simulink model "RotationalSolarPanelControl"  (R2022b)
settings: Solver=VariableStepAuto  StartTime=0.0  StopTime=15  RelTol=1e-3
undefined symbols (not defined in the file): J, Kd, Kf, Kg, Kt, R
libraries: slpidlib x1
settings Model: Creator=juan.moreira  LastModifiedBy=jprmj
settings ModelReferenceCC: EnableRefExpFcnMdlSchedulingChecks=on

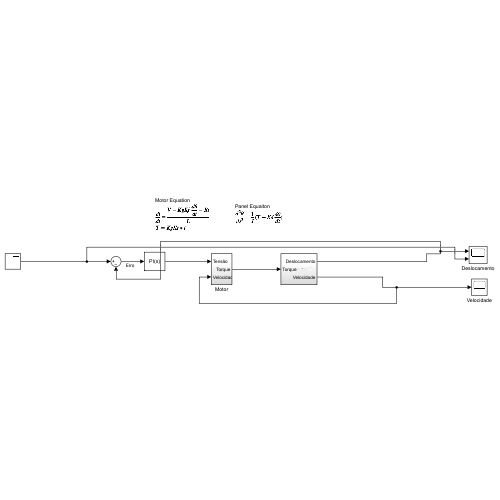
[thumbnail: Simulink's stored preview of the top-level diagram]
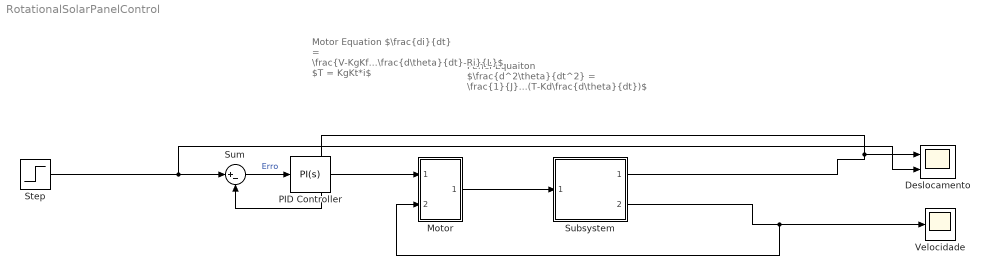
== system RotationalSolarPanelControl ==
  note: Panel Equaiton
      | $\frac{d^2\theta}{dt^2} = \frac{1}{J}(T-Kd\frac{d\theta}{dt})$
  note: Motor Equation
      | $\frac{di}{dt} = \frac{V-KgKf\frac{d\theta}{dt}-Ri}{L}$
      | $T = KgKt*i$
  Deslocamento : Scope  NumInputPorts=2
  Motor : Subsystem
  PID Controller : slpidlib/PID Controller  Controller=PI  Form=Parallel  TimeDomain=Continuous-time  UseExternalTs=off  SampleTime=-1  IntegratorMethod=Forward Euler  FilterMethod=Forward Euler  ControllerParametersSource=internal  P=180  I=140  UseKiTs=off  D=0  N=100  UseFilter=on  TunerSelectOption=Transfer Function Based (PID Tuner App)  InitialConditionSource=internal  InitialConditionForIntegrator=0  InitialConditionForFilter=0  DifferentiatorICPrevScaledInput=0  ExternalReset=none  TrackingMode=off  Kt=1  LimitOutput=off  SatLimitsSource=internal  UpperSaturationLimit=inf  LowerSaturationLimit=-inf  LinearizeAsGain=on  AntiWindupMode=none  Kb=1  LimitIntegrator=off  UpperIntegratorSaturationLimit=inf  LowerIntegratorSaturationLimit=-inf  POutMin=[]  POutMax=[]  IOutMin=[]  IOutMax=[]  DOutMin=[]  DOutMax=[]  NOutMin=[]  NOutMax=[]  SumOutMin=[]  SumOutMax=[]  SaturationOutMin=[]  SaturationOutMax=[]  PParamMin=[]  PParamMax=[]  IParamMin=[]  IParamMax=[]  DParamMin=[]  DParamMax=[]  NParamMin=[]  NParamMax=[]  KbParamMin=[]  KbParamMax=[]  KtParamMin=[]  KtParamMax=[]  KbOutMin=[]  KbOutMax=[]  KtOutMin=[]  KtOutMax=[]  IntegratorOutMin=[]  IntegratorOutMax=[]  FilterOutMin=[]  FilterOutMax=[]  SumI1OutMin=[]  SumI1OutMax=[]  SumI2OutMin=[]  SumI2OutMax=[]  SumI3OutMin=[]  SumI3OutMax=[]  SumI4OutMin=[]  SumI4OutMax=[]  SumDOutMin=[]  SumDOutMax=[]  DifferentiatorOutMin=[]  DifferentiatorOutMax=[]  FilterDiffOutCoefMin=[]  FilterDiffOutCoefMax=[]  ReciprocalOutMin=[]  ReciprocalOutMax=[]  SumDenOutMin=[]  SumDenOutMax=[]  SumNumOutMin=[]  SumNumOutMax=[]  DivideOutMin=[]  DivideOutMax=[]  UdiffTsProdOutMin=[]  UdiffTsProdOutMax=[]  NTsProdOutMin=[]  NTsProdOutMax=[]  UintegralTsProdOutMin=[]  UintegralTsProdOutMax=[]  UngainTsProdOutMin=[]  UngainTsProdOutMax=[]  ClampingZeroOutDataTypeStr=Inherit: Inherit via back propagation  ClampingZeroOutMin=[]  ClampingZeroOutMax=[]  FilterDenConstantOutDataTypeStr=Inherit: Inherit via back propagation  FilterDenConstantOutMin=[]  FilterDenConstantOutMax=[]  PCopyOutDataTypeStr=Inherit: Inherit via back propagation  PCopyOutMin=[]  PCopyOutMax=[]  NCopyOutDataTypeStr=Inherit: Inherit via back propagation  NCopyOutMin=[]  NCopyOutMax=[]  IntegratorContinuousStateAttributes=''  IntegratorStateMustResolveToSignalObject=off  IntegratorRTWStateStorageClass=Auto  FilterContinuousStateAttributes=''  FilterStateMustResolveToSignalObject=off  FilterRTWStateStorageClass=Auto  ParallelPVariant=InternalParameters  IdealPVariant=Disabled  IVariant=InternalParameters  DVariant=Disabled  IntegratorVariant=Continuous  SatVariant=Disabled  AWVariant=Passthrough  PCopyVariant=Disabled  TRVariant=Disabled  FdbkBlocksVariant=Forward  IdealPFdbkVariant=Disabled  SatFdbkVariant=Disabled  DerivativeFilterVariant=Disabled  NVariant=Disabled  NCopyVariant=Disabled_SignalSpec  FilterICVariant=Disabled  IntegratorICVariant=InternalICs  ExternalResetVariant=Disabled  TRSumVariant=Passthrough  SumFdbkVariant=Disabled  SumVariant=Sum_PI  TsampFilterVariant=InternalTs  TsampNgainVariant=Passthrough  TsampIntegralVariant=Passthrough  ExternalSaturationOutDataTypeStr=Inherit: Same as second input
  Step : Step  SampleTime=0
  Subsystem : Subsystem
  Sum : Sum  Inputs=|+-
  Velocidade : Scope
  wires:
  Subsystem/2(Velocidade) -> Motor/2(Velocidade), Velocidade/1
  Subsystem/1(Deslocamento) -> Sum/2, Deslocamento/1
  Motor/1(Torque) -> Subsystem/1(Torque)
  Step/1 -> Deslocamento/2, Sum/1
  Sum/1 -> PID Controller/1  "Erro"
  PID Controller/1 -> Motor/1(Tensão)

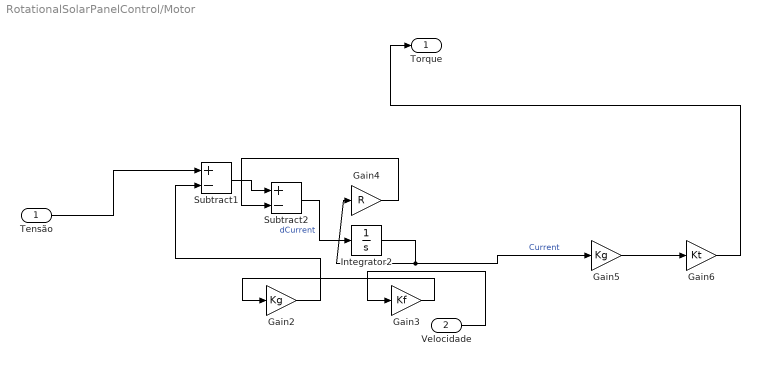
== system RotationalSolarPanelControl/Motor ==
  Tensão : Inport
  Velocidade : Inport  Port=2
  Gain2 : Gain  Gain=Kg
  Gain3 : Gain  Gain=Kf
  Gain4 : Gain  Gain=R
  Gain5 : Gain  Gain=Kg
  Gain6 : Gain  Gain=Kt
  Integrator2 : Integrator
  Subtract1 : Sum  Inputs=+-
  Subtract2 : Sum  Inputs=+-
  Torque : Outport
  wires:
  Gain2/1 -> Subtract1/2
  Gain3/1 -> Gain2/1
  Velocidade/1 -> Gain3/1
  Integrator2/1 -> Gain5/1, Gain4/1  "Current"
  Gain4/1 -> Subtract2/2
  Subtract2/1 -> Integrator2/1  "dCurrent"
  Subtract1/1 -> Subtract2/1
  Gain5/1 -> Gain6/1
  Gain6/1 -> Torque/1
  Tensão/1 -> Subtract1/1

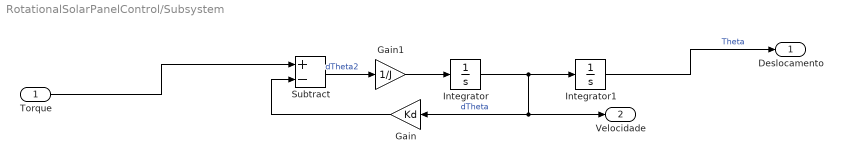
== system RotationalSolarPanelControl/Subsystem ==
  Torque : Inport
  Gain : Gain  Gain=Kd
  Gain1 : Gain  Gain=1/J
  Integrator : Integrator
  Integrator1 : Integrator
  Subtract : Sum  Inputs=+-
  Deslocamento : Outport
  Velocidade : Outport  Port=2
  wires:
  Gain/1 -> Subtract/2
  Integrator/1 -> Integrator1/1, Velocidade/1, Gain/1  "dTheta"
  Subtract/1 -> Gain1/1  "dTheta2"
  Gain1/1 -> Integrator/1
  Torque/1 -> Subtract/1
  Integrator1/1 -> Deslocamento/1  "Theta"
